simulink model "task_B2_mod"  (R2013b)
settings: Solver=ode45  StartTime=0.0  StopTime=10.0  RelTol=1e-3
values from neighbouring files (symbols this model uses):
  a0 = 8*lamda/(c*ro*(b-a)^2)    [task_A_scr.m]    (also in task_B_scr.m = 8*lamda/(3*c*ro*(b-a)^2); task_C_scr.m = 4*lamda*(2-A1-B1)/(c*ro*(b-a)^2))
  b0 = a0/2    [task_A_scr.m]    (also in task_B_scr.m)
  q_a = 500000    [task_B_scr.m]
  T_b = 400    [task_A_scr.m]    (also in task_B_scr.m = 350; task_C_scr.m = 300)
undefined symbols (not defined in the file or in its folder): a, b, lamda, T_0
settings Model: Creator=Yurii  LastModifiedBy=Yurii

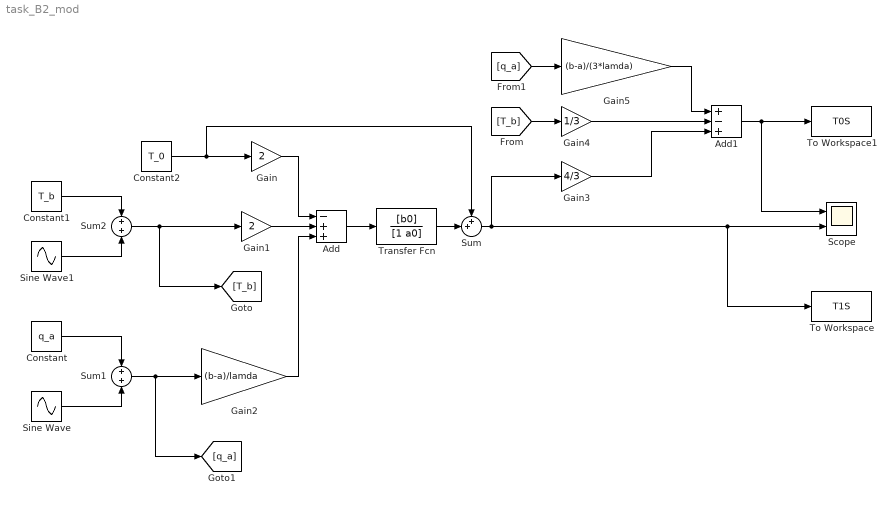
== system task_B2_mod ==
  Add : Sum  Inputs=-++
  Add1 : Sum  Inputs=+-+
  Constant : Constant  Value=q_a
  Constant1 : Constant  Value=T_b
  Constant2 : Constant  Value=T_0
  Gain : Gain  Gain=2
  Gain1 : Gain  Gain=2
  Gain2 : Gain  Gain=(b-a)/lamda
  Gain3 : Gain  Gain=4/3
  Gain4 : Gain  Gain=1/3
  Gain5 : Gain  Gain=(b-a)/(3*lamda)
  Scope : Scope  NumInputPorts=2
      settings: YMin=-5~-5  YMax=5~5
  Sine Wave : Sin  Amplitude=0.05*q_a  SampleTime=0
  Sine Wave1 : Sin  Amplitude=0.05*T_b  SampleTime=0
  Sum : Sum  Inputs=++|
  Sum1 : Sum  Inputs=+|+
  Sum2 : Sum  Inputs=+|+
  To Workspace : ToWorkspace  VariableName=T1S  SampleTime=-1  SaveFormat=Timeseries
  To Workspace1 : ToWorkspace  VariableName=T0S  SampleTime=-1  SaveFormat=Timeseries
  Transfer Fcn : TransferFcn  Numerator=[b0]  Denominator=[1 a0]
  wires:
  Constant2/1 -> Gain/1, Sum/1
  Gain/1 -> Add/1
  Add/1 -> Transfer Fcn/1
  Transfer Fcn/1 -> Sum/2
  Sum/1 -> To Workspace/1, Scope/2, Gain3/1
  Gain1/1 -> Add/2
  Gain2/1 -> Add/3
  [T_b] -> Gain4/1
  [q_a] -> Gain5/1
  Gain4/1 -> Add1/2
  Gain5/1 -> Add1/1
  Gain3/1 -> Add1/3
  Add1/1 -> To Workspace1/1, Scope/1
  Constant/1 -> Sum1/1
  Sine Wave/1 -> Sum1/2
  Sum1/1 -> [q_a], Gain2/1
  Sine Wave1/1 -> Sum2/2
  Constant1/1 -> Sum2/1
  Sum2/1 -> [T_b], Gain1/1
